simulink model "partial_acc_model_resilient"  (Simulink 8.9)
settings: Solver=VariableStepAuto  StartTime=0.0  StopTime=Tsim  RelTol=1e-3
values from neighbouring files (symbols this model uses):
  d0 = 50    [acc_execution.m]    (also in acc_muti.m = 100)
  ed0 = d0    (= 50)    [acc_execution.m]    (also in acc_muti.m = 1)
  ev0 = v0    (= 25)    [acc_execution.m]    (also in acc_muti.m = 1)
  nrad = 0    [acc_execution.m]    (also in acc_muti.m)
  v0 = 25    [acc_execution.m]    (also in acc_muti.m)
  vl = 20    [acc_execution.m]    (also in acc_muti.m = 26)
settings Model: Creator=LuanNguyen  LastModifiedBy=LuanNguyen
settings DataIOCC: LimitDataPoints=off  SaveFormat=Dataset  SignalLoggingSaveFormat=Dataset
settings OptimizationCC: LifeSpan=auto
settings DebuggingCC: UnderspecifiedInitializationDetection=Simplified  MergeDetectMultiDrivingBlocksExec=error  FcnCallInpInsideContextMsg=error  StateNameClashWarn=none  SFUnexpectedBacktrackingDiag=error  SFNoUnconditionalDefaultTransitionDiag=error  SFExecutionAtInitializationDiag=warning
settings HardwareCC: ProdBitPerPointer=64  ProdBitPerSizeT=64  ProdBitPerPtrDiffT=64  ProdLargestAtomicFloat=Float  ProdIntDivRoundTo=Zero  ProdEndianess=LittleEndian  ProdWordSize=64  ProdHWDeviceType=Intel->x86-64 (Windows64)
settings ModelReferenceCC: PropagateSignalLabelsOutOfModel=on
settings GRTTargetCC: TargetLangStandard=C99 (ISO)  GeneratePreprocessorConditionals=Use local settings  CombineOutputUpdateFcns=on  GRTInterface=off
settings ConfigComp: CovMetricSettings=dwe  CovHtmlReporting=off  CovSaveCumulativeToWorkspaceVar=off  CovSaveSingleToWorkspaceVar=off  CovExternalEMLEnable=on

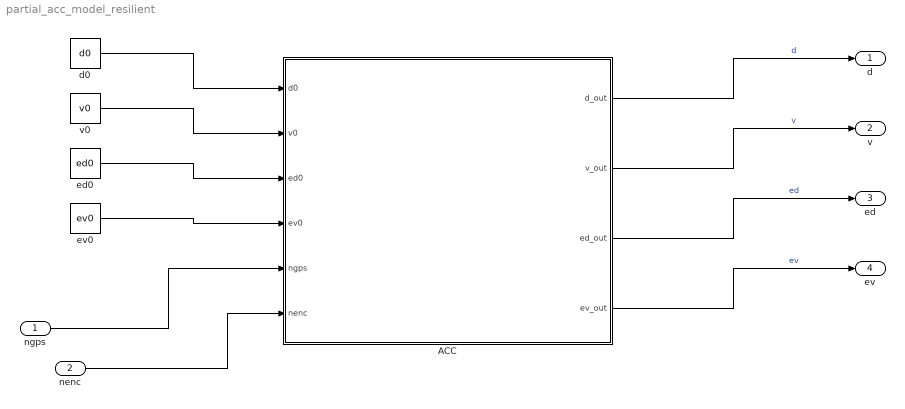
== system partial_acc_model_resilient ==
  ngps : Inport
  nenc : Inport  Port=2
  ACC : Stateflow chart  TreatAsAtomicUnit=on
  d0 : Constant  Value=d0
  ed0 : Constant  Value=ed0
  ev0 : Constant  Value=ev0
  v0 : Constant  Value=v0
  d : Outport
  v : Outport  Port=2
  ed : Outport  Port=3
  ev : Outport  Port=4
  wires:
  ACC/1(d_out) -> d/1  "d"
  ACC/2(v_out) -> v/1  "v"
  ACC/3(ed_out) -> ed/1  "ed"
  ACC/4(ev_out) -> ev/1  "ev"
  d0/1 -> ACC/1(d0)
  v0/1 -> ACC/2(v0)
  ed0/1 -> ACC/3(ed0)
  ev0/1 -> ACC/4(ev0)
  ngps/1 -> ACC/5(ngps)
  nenc/1 -> ACC/6(nenc)

== stateflow chart ACC ==
  settings: updateMethod=CONTINUOUS
  state Spacing_Control
    du:
    d_dot = -v+vl;
    v_dot = 0.25*d - 2*v - 0.25*ed + ev - 0.25*(10 + 2*(v-ev))+2*vl;
    ed_dot = -10*ed - ev + nrad;
    ev_dot = -2*ev+0.5*(ngps + nenc);
    d_out = d;
    v_out = v;
    ed_out = ed;
    ev_out = ev;
  state Speed_Control
    du:
    d_dot = -v+vl;
    v_dot = -2*v+ev+2*vl;
    ed_dot = -10*ed - ev + nrad;
    ev_dot = -2*ev+0.5*(ngps + nenc);
    d_out = d;
    v_out = v;
    ed_out = ed;
    ev_out = ev;
  state Spacing_Control_Resilient
    du:
    d_dot = -v+vl;
    v_dot = 0.25*d - 2*v - 0.25*ed + ev - 0.25*(10 + 2*(v-ev))+2*vl;
    ed_dot = -10*ed - ev + nrad;
    ev_dot = -2*ev+0.5*(0 + nenc);
    d_out = d;
    v_out = v;
    ed_out = ed;
    ev_out = ev;
  state Speed_Control_Resilient
    du:
    d_dot = -v+vl;
    v_dot = -2*v+ev+2*vl;
    ed_dot = -10*ed - ev + nrad;
    ev_dot = -2*ev+0.5*(0 + nenc);
    d_out = d;
    v_out = v;
    ed_out = ed;
    ev_out = ev;
  (default) -> Speed_Control : {d = d0; v = v0; ed = ed0; ev = ev0;}
  Spacing_Control_Resilient -> Spacing_Control [order 2] : [abs(ngps-nenc) <8]
  Speed_Control_Resilient -> Speed_Control [order 2] : [abs(ngps-nenc) <8]
  Speed_Control -> Spacing_Control [order 1] : [d - ed < 10 + 2*(v-ev)]
  Spacing_Control -> Speed_Control [order 1] : [d - ed >= 10 + 2*(v-ev)]
  Speed_Control -> Speed_Control_Resilient [order 2] : [abs(ngps-nenc) >9]
  Spacing_Control -> Spacing_Control_Resilient [order 2] : [abs(ngps-nenc) >9]
  Speed_Control_Resilient -> Spacing_Control_Resilient [order 1] : [d - ed < 10 + 2*(v-ev)]
  Spacing_Control_Resilient -> Speed_Control_Resilient [order 1] : [d - ed >= 10 + 2*(v-ev)]
  data: ed local double; ev local double; v local double; d_out output double; v_out output double; ed_out output double; ev_out output double; vl local double; nrad local double; d0 input double; v0 input double; ed0 input double; ev0 input double; d local double; ngps input double; nenc input double
  data ed settings: updateMethod=SF_CONTINUOUS_TIME_DATA
  data ev settings: updateMethod=SF_CONTINUOUS_TIME_DATA
  data v settings: updateMethod=SF_CONTINUOUS_TIME_DATA
  data d settings: updateMethod=SF_CONTINUOUS_TIME_DATA
